simulink model "send_UE"  (R2016a)
settings: Solver=FixedStepAuto  StartTime=0.0  StopTime=inf  RelTol=1e-3
libraries: dspsigops x1, aerolibanimutils x1
settings Model: Creator=Florian Wachter  LastModifiedBy=Florian Wachter

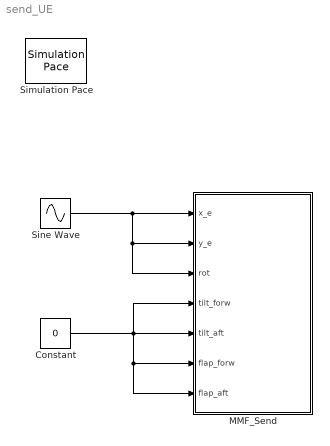
== system send_UE ==
  Constant : Constant  Value=0
  MMF_Send : Subsystem
  Simulation Pace : aerolibanimutils/Simulation Pace  SimulationPace=1  SleepMode=MATLAB Thread  OutputPaceError=off  SampleTime=1/30
  Sine Wave : Sin  Amplitude=5  Bias=5  Frequency=2  SampleTime=0
  wires:
  Sine Wave/1 -> MMF_Send/1(x_e), MMF_Send/2(y_e), MMF_Send/3(rot)
  Constant/1 -> MMF_Send/4(tilt_forw), MMF_Send/5(tilt_aft), MMF_Send/7(flap_aft), MMF_Send/6(flap_forw)

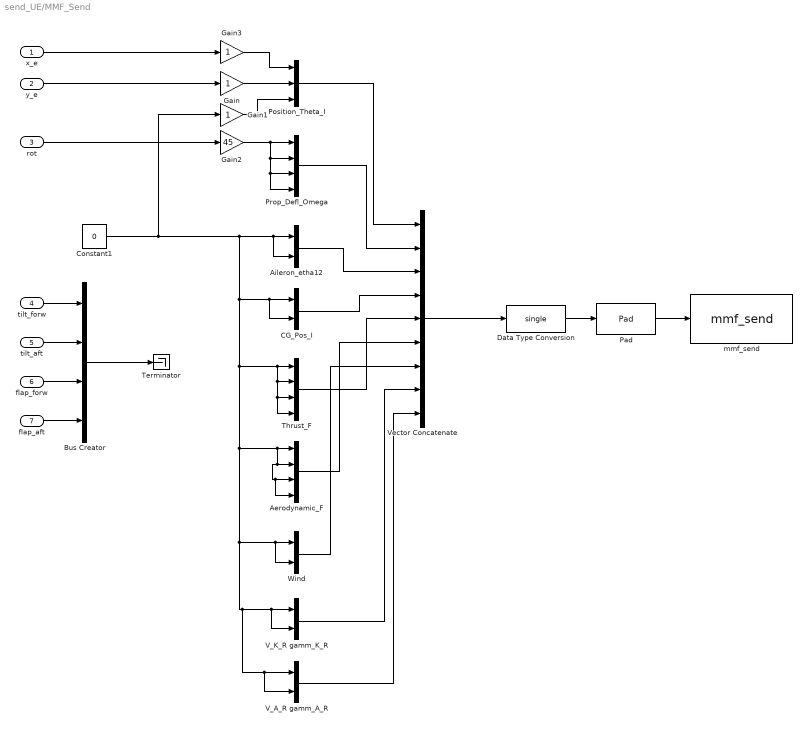
== system send_UE/MMF_Send ==
  x_e : Inport
  y_e : Inport  Port=2
  rot : Inport  Port=3
  tilt_forw : Inport  Port=4
  tilt_aft : Inport  Port=5
  flap_forw : Inport  Port=6
  flap_aft : Inport  Port=7
  Aerodynamic_F : Concatenate  NumInputs=4
  Aileron_etha12 : Concatenate
  Bus Creator : BusCreator  Inputs=4
  CG_Pos_I : Concatenate
  Constant1 : Constant  Value=0
  Data Type Conversion : DataTypeConversion  OutMax=[100]  OutDataTypeStr=single
  Gain : Gain
  Gain1 : Gain
  Gain2 : Gain  Gain=45
  Gain3 : Gain
  Pad : dspsigops/Pad  padAlong=Rows  dimsToPad=1  valSrc=Specify via dialog  padVal=0  spec=Output size  padNumOutRowsSpecMethod=User-specified  numOutRows=1  padNumOutColsSpecMethod=User-specified  numOutCols=100  isVarDimsMode=off  padBeginning=0  padEnd=0  outSizeMode=User-specified  outSize=1  padSigAt=End  trunc_flag=None  roundingMode=Floor  overflowMode=off  truncOrWrapMode=Truncate  wrap_flag=None
  Position_Theta_I : Concatenate  NumInputs=3
  Prop_Defl_Omega : Concatenate  NumInputs=4
  Terminator : Terminator
  Thrust_F : Concatenate  NumInputs=4
  V_A_R gamm_A_R : Concatenate
  V_K_R gamm_K_R : Concatenate
  Vector Concatenate : Concatenate  NumInputs=9
  Wind : Concatenate
  mmf_send : S-Function  FunctionName=mmf_send  SFunctionDeploymentMode=off  EnableBusSupport=off  mask(Legacy Function){SFunctionSpec=void mmf_send(single u1[100]), ShowSpec=on}
      mask prompts: ShowSpec "Display function specification"
      mask help:
      | This block allows you to call the legacy functions specified by the following Legacy Code Tool definition:
      | def.SFunctionName = 'mmf_send';
      | def.OutputFcnSpec = 'void mmf_send(single u1[100])';
      | def.StartFcnSpec = 'mmf_init()';
      | def.TerminateFcnSpec = 'mmf_close()';
      | def.HeaderFiles = {'mmf_send_dll.h'};
      | def.HostLibFiles = {'mmf_send_dll.lib'};
      mask Help: <p>This block was generated automatically by the Legacy Code Tool. For detailed help on this tool, call<a href="matlab:legacy_code('help')"> legacy_code('help')</a>.</p>
      mask Callback ShowSpec:
      | if strcmp(get_param(gcbh, 'ShowSpec'), 'on')
      |   set_param(gcbh, 'MaskDisplay', sprintf('fprintf(''%s'');', get_param(gcbh, 'SFunctionSpec')));
      | else
      |   set_param(gcbh, 'MaskDisplay', sprintf('fprintf(''%s'');', get_param(gcbh, 'FunctionName')));
      | end
      mask Display: fprintf('void mmf_send(single u1[100])');
  wires:
  Data Type Conversion/1 -> Pad/1
  Vector Concatenate/1 -> Data Type Conversion/1
  Position_Theta_I/1 -> Vector Concatenate/1
  Prop_Defl_Omega/1 -> Vector Concatenate/2
  Aileron_etha12/1 -> Vector Concatenate/3
  CG_Pos_I/1 -> Vector Concatenate/4
  Thrust_F/1 -> Vector Concatenate/5
  Aerodynamic_F/1 -> Vector Concatenate/6
  Wind/1 -> Vector Concatenate/7
  V_K_R gamm_K_R/1 -> Vector Concatenate/8
  V_A_R gamm_A_R/1 -> Vector Concatenate/9
  Constant1/1 -> Gain1/1, V_A_R gamm_A_R/2, V_A_R gamm_A_R/1, V_K_R gamm_K_R/2, V_K_R gamm_K_R/1, Wind/2, Wind/1, Aerodynamic_F/4, Aerodynamic_F/3, Aerodynamic_F/2, Aerodynamic_F/1, Thrust_F/4, Thrust_F/3, Thrust_F/2, Thrust_F/1, CG_Pos_I/2, CG_Pos_I/1, Aileron_etha12/2, Aileron_etha12/1
  Pad/1 -> mmf_send/1
  Gain/1 -> Position_Theta_I/2
  Gain1/1 -> Position_Theta_I/3
  Gain2/1 -> Prop_Defl_Omega/4, Prop_Defl_Omega/3, Prop_Defl_Omega/2, Prop_Defl_Omega/1
  Gain3/1 -> Position_Theta_I/1
  tilt_forw/1 -> Bus Creator/1
  flap_forw/1 -> Bus Creator/3
  x_e/1 -> Gain3/1
  y_e/1 -> Gain/1
  tilt_aft/1 -> Bus Creator/2
  flap_aft/1 -> Bus Creator/4
  Bus Creator/1 -> Terminator/1
  rot/1 -> Gain2/1
